simulink model "CH13_1"  (Simulink 7.5)
settings: Solver=ode45  StartTime=0.0  StopTime=0.001  RelTol=1e-3
libraries: dsparch4 x1, commsynccomp2 x1
settings Model: Creator=my2  LastModifiedBy=xnote
settings OptimizationCC: ExpressionDepthLimit=128
settings DebuggingCC: MultiTaskDSMMsg=warning  MultiTaskCondExecSysMsg=none  StateNameClashWarn=none
settings RTWCC: IncludeERTFirstTime=on
settings CodeAppCC: CustomSymbolStrType=$N$R$M_T
settings GRTTargetCC: CombineOutputUpdateFcns=on  CPPClassGenCompliant=on

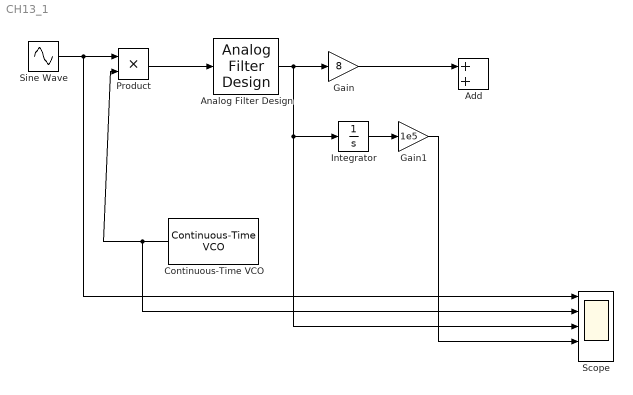
== system CH13_1 ==
  Add : Sum
  Analog Filter Design : dsparch4/Analog Filter Design  method=Chebyshev II  filttype=Lowpass  N=32  Wlo=30  Whi=80  Rp=2  Rs=40
  Continuous-Time VCO : commsynccomp2/Continuous-Time VCO  SystemSampleTime=-1  Ac=1  Fc=10  Kc=1  Ph=0
  Gain : Gain  Gain=8
  Gain1 : Gain  Gain=1e5
  Integrator : Integrator
  Product : Product
  Scope : Scope  NumInputPorts=5
      settings: YMin=-5~-5~-5~-5~-5  YMax=5~5~5~5~5
  Sine Wave : Sin  Amplitude=1  Bias=0  Frequency=1  Phase=0  Samples=10  SampleTime=0  Offset=0
  wires:
  Product/1 -> Analog Filter Design/1
  Analog Filter Design/1 -> Scope/3, Integrator/1, Gain/1
  Integrator/1 -> Gain1/1
  Gain/1 -> Add/1
  Gain1/1 -> Scope/4
  Continuous-Time VCO/1 -> Scope/2, Product/2
  Sine Wave/1 -> Scope/1, Product/1
